simulink model "UDP_Simulink_Tst"  (R2022a)
settings: Solver=ode4  StartTime=0.0  StopTime=inf  FixedStep=1/1000  RelTol=1e-3
libraries: dspnetwork x1
settings Model: SimulationMode=accelerator  Creator=Fatabi  LastModifiedBy=Fatabi

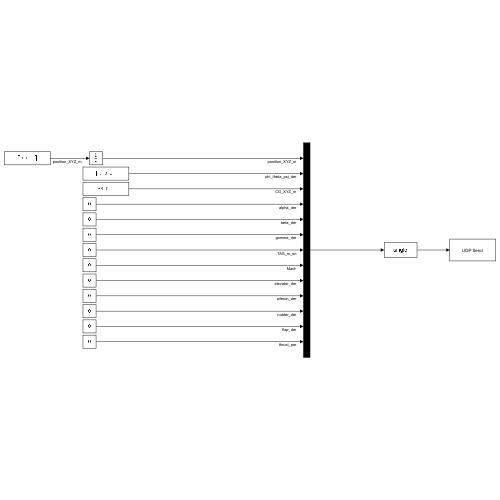
[thumbnail: Simulink's stored preview of the top-level diagram]
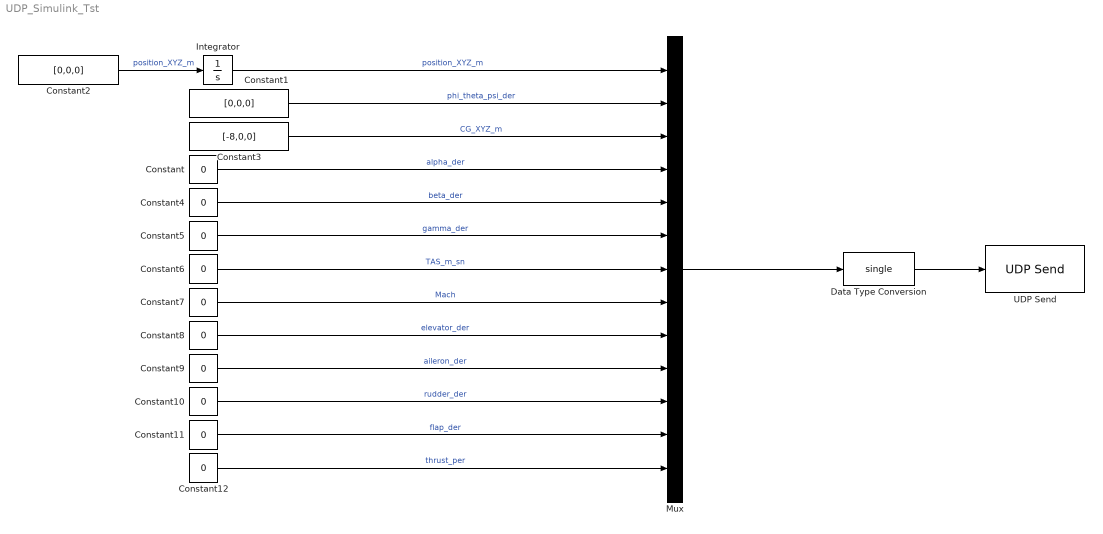
== system UDP_Simulink_Tst ==
  Constant{,4..12} (10 alike) : Constant  Value=0
  Constant1 : Constant  Value=[0,0,0]
  Constant2 : Constant  Value=[0,0,0]
  Constant3 : Constant  Value=[-8,0,0]
  Data Type Conversion : DataTypeConversion  OutDataTypeStr=single  SaturateOnIntegerOverflow=off  RndMeth=Floor
  Integrator : Integrator
  Mux : Mux  Inputs=13
  UDP Send : dspnetwork/UDP Send  remoteURL='127.0.0.1'  remotePort=8001  localURL='0.0.0.0'  localPortSource=Automatically determine  localPort=-1  sendBufferSize=76  sampletime=-1  blockPlatform=[]  separateLengthPort=0
  wires:
  Constant9/1 -> Mux/10  "aileron_der"
  Constant5/1 -> Mux/6  "gamma_der"
  Constant11/1 -> Mux/12  "flap_der"
  Constant/1 -> Mux/4  "alpha_der"
  Constant10/1 -> Mux/11  "rudder_der"
  Constant4/1 -> Mux/5  "beta_der"
  Constant3/1 -> Mux/3  "CG_XYZ_m"
  Constant8/1 -> Mux/9  "elevator_der"
  Data Type Conversion/1 -> UDP Send/1
  Mux/1 -> Data Type Conversion/1
  Constant1/1 -> Mux/2  "phi_theta_psi_der"
  Constant6/1 -> Mux/7  "TAS_m_sn"
  Constant7/1 -> Mux/8  "Mach"
  Constant12/1 -> Mux/13  "thrust_per"
  Integrator/1 -> Mux/1  "position_XYZ_m"
  Constant2/1 -> Integrator/1  "position_XYZ_m"
